simulink model "D6"  (R2017b)
settings: Solver=VariableStepAuto  StartTime=0.0  StopTime=700  RelTol=1e-3
libraries: simulink x3
settings Model: Creator=frank  LastModifiedBy=frank
settings SolverCC: ZeroCrossAlgorithm=Adaptive

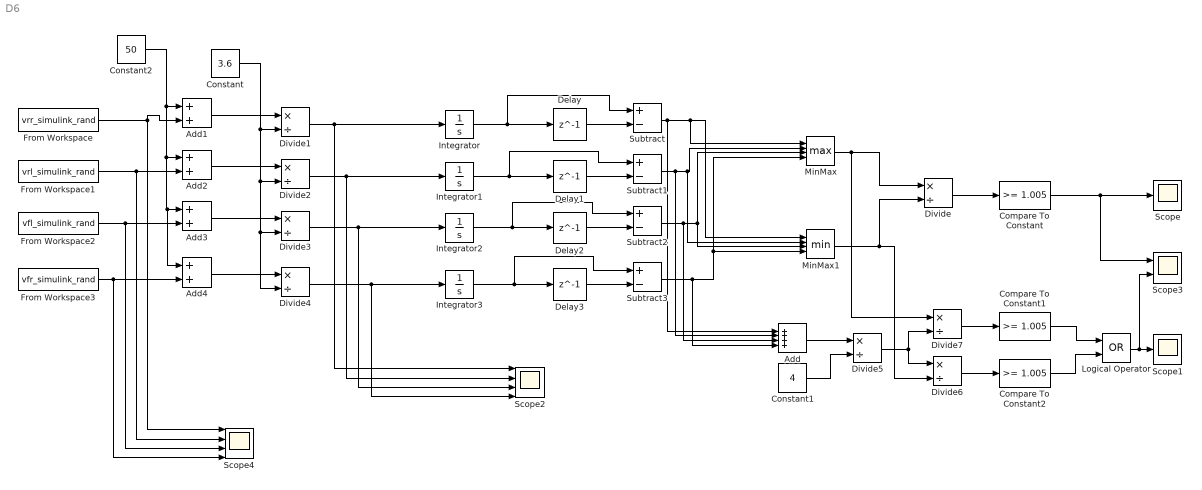
== system D6 ==
  Add : Sum  Inputs=4
  Add{1..4} (4 alike) : Sum
  Compare To Constant : simulink/Logic and Bit Operations/Compare To Constant  relop=>=  const=1.005  OutDataTypeStr=boolean
  Compare To Constant1 : simulink/Logic and Bit Operations/Compare To Constant  relop=>=  const=1.005  OutDataTypeStr=boolean
  Compare To Constant2 : simulink/Logic and Bit Operations/Compare To Constant  relop=>=  const=1.005  OutDataTypeStr=boolean
  Constant : Constant  Value=3.6
  Constant1 : Constant  Value=4
  Constant2 : Constant  Value=50
  Delay{,1..3} (4 alike) : Delay  DelayLength=1  InitialCondition=0  SampleTime=10
  Divide{,1..7} (8 alike) : Product  Inputs=*/
  From Workspace : FromWorkspace  VariableName=vrr_simulink_rand  SampleTime=0
  From Workspace1 : FromWorkspace  VariableName=vrl_simulink_rand  SampleTime=0
  From Workspace2 : FromWorkspace  VariableName=vfl_simulink_rand  SampleTime=0
  From Workspace3 : FromWorkspace  VariableName=vfr_simulink_rand  SampleTime=0
  Integrator{,1..3} (4 alike) : Integrator
  Logical Operator : Logic  Operator=OR  AllPortsSameDT=off  OutDataTypeStr=boolean
  MinMax : MinMax  Function=max  Inputs=4
  MinMax1 : MinMax  Inputs=4
  Scope : Scope
  Scope1 : Scope
  Scope2 : Scope  NumInputPorts=4
  Scope3 : Scope  NumInputPorts=2
  Scope4 : Scope  NumInputPorts=4
  Subtract{,1..3} (4 alike) : Sum  Inputs=+-
  wires:
  Divide1/1 -> Scope2/1, Integrator/1
  Divide2/1 -> Scope2/2, Integrator1/1
  Divide3/1 -> Scope2/3, Integrator2/1
  Divide4/1 -> Scope2/4, Integrator3/1
  Constant/1 -> Divide4/2, Divide3/2, Divide2/2, Divide1/2
  Integrator/1 -> Subtract/1, Delay/1
  Integrator1/1 -> Subtract1/1, Delay1/1
  Integrator2/1 -> Subtract2/1, Delay2/1
  Integrator3/1 -> Subtract3/1, Delay3/1
  Delay/1 -> Subtract/2
  Delay3/1 -> Subtract3/2
  Delay2/1 -> Subtract2/2
  Delay1/1 -> Subtract1/2
  Subtract/1 -> Add/1, MinMax1/1, MinMax/1
  Subtract1/1 -> Add/2, MinMax1/2, MinMax/2
  Subtract3/1 -> Add/4, MinMax1/4, MinMax/4
  MinMax/1 -> Divide7/1, Divide/1
  MinMax1/1 -> Divide6/2, Divide/2
  Divide/1 -> Compare To Constant/1
  Compare To Constant/1 -> Scope3/1, Scope/1
  Subtract2/1 -> Add/3, MinMax1/3, MinMax/3
  Add/1 -> Divide5/1
  Constant1/1 -> Divide5/2
  Divide5/1 -> Divide6/1, Divide7/2
  Divide7/1 -> Compare To Constant1/1
  Divide6/1 -> Compare To Constant2/1
  Compare To Constant1/1 -> Logical Operator/1
  Compare To Constant2/1 -> Logical Operator/2
  Logical Operator/1 -> Scope3/2, Scope1/1
  From Workspace/1 -> Add1/2, Scope4/1
  Add1/1 -> Divide1/1
  From Workspace1/1 -> Scope4/2, Add2/2
  Add2/1 -> Divide2/1
  From Workspace2/1 -> Scope4/3, Add3/2
  Add3/1 -> Divide3/1
  From Workspace3/1 -> Scope4/4, Add4/2
  Add4/1 -> Divide4/1
  Constant2/1 -> Add4/1, Add3/1, Add2/1, Add1/1
